simulink model "animation"  (R2023b)
settings: Solver=VariableStepAuto  StartTime=0.0  StopTime=30  RelTol=1e-3
libraries: vrlib x3, simulink x1
settings Model: Creator=tinas  LastModifiedBy=tinas

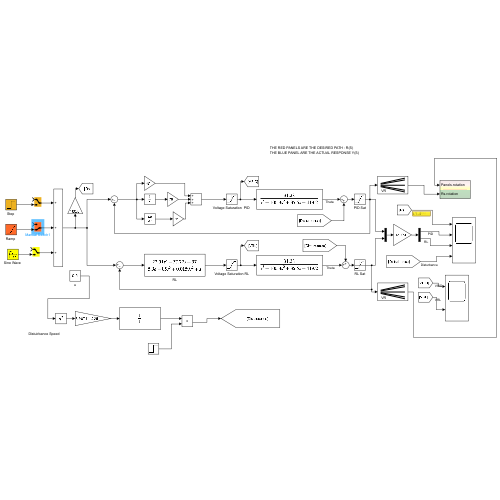
[thumbnail: Simulink's stored preview of the top-level diagram]
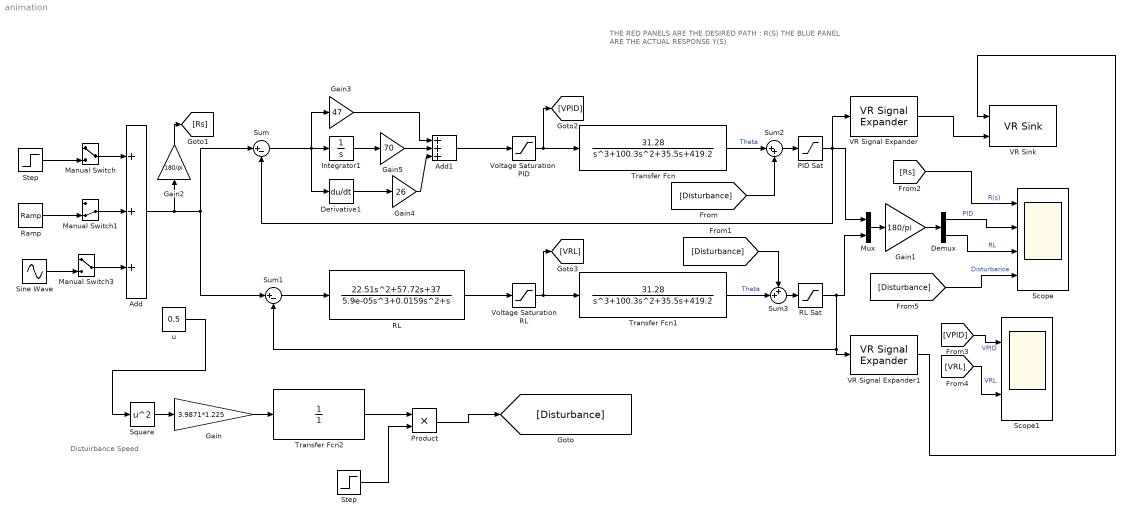
== system animation ==
  note: Distuirbance Speed
  note: THE RED PANELS ARE THE DESIRED PATH : R(S)
      | THE BLUE PANEL ARE THE ACTUAL RESPONSE Y(S)
  Add : Sum  Inputs=+++
  Add1 : Sum  Inputs=+++
  Demux : Demux  Outputs=2
  Derivative1 : Derivative
  Gain : Gain  Gain=3.9871*1.225
  Gain1 : Gain  Gain=180/pi
  Gain2 : Gain  Gain=180/pi
  Gain3 : Gain  Gain=47
  Gain4 : Gain  Gain=26
  Gain5 : Gain  Gain=70
  Integrator1 : Integrator
  Manual Switch : ManualSwitch
  Manual Switch1 : ManualSwitch  CurrentSetting=0
  Manual Switch3 : ManualSwitch
  Mux : Mux  Inputs=2
  PID Sat : Saturate  UpperLimit=pi/2  LowerLimit=-pi/2
  Product : Product
  RL : TransferFcn  Numerator=[22.51 57.72 37 ]  Denominator="[5.9e-05  0.0159  1 0]"
  RL Sat : Saturate  UpperLimit=pi/2  LowerLimit=-pi/2
  "Ramp " : simulink/Sources/Ramp  slope=0.01  start=0  InitialOutput=0
  Scope : Scope  NumInputPorts=4
  Scope1 : Scope  NumInputPorts=2
  "Sine Wave " : Sin  Amplitude=pi/2  SampleTime=0
  Square : Math  Operator=square
  Step : Step  Time=10  SampleTime=0
  "Step " : Step  Time=0  After=45*pi/180  SampleTime=0
  Sum : Sum  Inputs=|+-
  Sum1 : Sum  Inputs=|+-
  Sum2 : Sum  Inputs=|++
  Sum3 : Sum  Inputs=++|
  Transfer Fcn : TransferFcn  Numerator=[31.28]  Denominator="[1 100.3  35.5 419.2]"
  Transfer Fcn1 : TransferFcn  Numerator=[31.28]  Denominator="[1 100.3  35.5 419.2]"
  Transfer Fcn2 : TransferFcn  Denominator=[1]
  VR Signal Expander : vrlib/VR Signal Expander  outwidth=4  outidx=[4]
  VR Signal Expander1 : vrlib/VR Signal Expander  outwidth=4  outidx=[4]
  VR Sink : vrlib/VR Sink  InstantiateOnLoad=on  SampleTime=0.1  ViewEnable=on  RemoteChange=off  RemoteView=off  FieldsWritten=Panels.rotation.4.1.1.double#Rs.rotation.4.1.1.double  WorldFileName=Solar_Tracker.x3d  AutoView=off  VideoDimensions=[]  AllowVariableSize=off  FigureProperties="{'Position', 'Name', 'Viewpoint', 'CameraBound', 'CameraDirection', 'CameraPosition', 'CameraUpVector', 'ZoomFactor', 'Antialiasing', 'Headlight', 'Lighting', 'NavPanel', 'Sound', 'StatusBar', 'Stereo3D', 'Stereo3DCameraOffset', 'Stereo3DHIT', 'ToolBar', 'Textures', 'Transparency', 'Triad', 'Wireframe', 'NavZones', 'NavMode', 'NavSpeed', 'CaptureFileFormat', 'CaptureFileName', 'Record2DCompressMethod', 'Record2DCompressQuality', 'Record2D', 'Record2DFileName', 'Record2DFPS'; [6.2900000000000000e+02  -4.5540000000000009e+02   5.7600000000000000e+02   3.5000000000000000e+02], '', '', 'on', [0.0000000000000000e+00   0.0000000000000000e+00  -1.0000000000000000e+00], [0.0000000000000000e+00   0.0000000000000000e+00   1.0000000000000000e+01], [0.0000000000000000e+00   1.0000000000000000e+00   0.0000000000000000e+00], [2.5937424601000023e+00], 'on', 'on', 'on', 'halfbar', 'on', 'on', 'off', [1.0000000149011612e-01], [0.0000000000000000e+00], 'on', 'on', 'on', 'none', 'off', 'off', 'fly', 'normal', 'tif', '%f_anim_%n.tif', 'auto', [7.5000000000000000e+01], 'off', '%f_anim_%n.avi', 'auto'}"
  "Voltage Saturation  PID " : Saturate  UpperLimit=230  LowerLimit=-230
  Voltage Saturation RL : Saturate  UpperLimit=230  LowerLimit=-230
  u : Constant  Value=0.5
  wires:
  "Sine Wave "/1 -> Manual Switch3/2
  "Step "/1 -> Manual Switch/2
  Manual Switch3/1 -> Add/3
  Manual Switch1/1 -> Add/2
  "Ramp "/1 -> Manual Switch1/2
  Manual Switch/1 -> Add/1
  Add/1 -> Gain2/1, Sum1/1, Sum/1
  "Voltage Saturation  PID "/1 -> [VPID], Transfer Fcn/1
  Voltage Saturation RL/1 -> [VRL], Transfer Fcn1/1
  Add1/1 -> "Voltage Saturation  PID "/1
  Gain3/1 -> Add1/1
  Derivative1/1 -> Gain4/1
  Gain4/1 -> Add1/3
  Gain5/1 -> Add1/2
  Integrator1/1 -> Gain5/1
  Sum/1 -> Gain3/1, Derivative1/1, Integrator1/1
  RL/1 -> Voltage Saturation RL/1
  Sum1/1 -> RL/1
  u/1 -> Square/1
  Square/1 -> Gain/1
  Gain/1 -> Transfer Fcn2/1
  [Disturbance] -> Sum2/2
  [Disturbance] -> Sum3/1
  Mux/1 -> Gain1/1
  Gain2/1 -> [Rs]
  [Rs] -> Scope/1  "R(s)"
  Gain1/1 -> Demux/1
  Demux/1 -> Scope/2  "PID"
  Demux/2 -> Scope/3  "RL"
  [VRL] -> Scope1/2  "VRL"
  [VPID] -> Scope1/1  "VPID"
  [Disturbance] -> Scope/4  "Disturbance"
  Transfer Fcn2/1 -> Product/1
  Step/1 -> Product/2
  Product/1 -> [Disturbance]
  Transfer Fcn/1 -> Sum2/1  "Theta"
  Sum2/1 -> PID Sat/1
  PID Sat/1 -> VR Signal Expander/1, Sum/2, Mux/1
  Transfer Fcn1/1 -> Sum3/2  "Theta"
  Sum3/1 -> RL Sat/1
  RL Sat/1 -> VR Signal Expander1/1, Sum1/2, Mux/2
  VR Signal Expander/1 -> VR Sink/2
  VR Signal Expander1/1 -> VR Sink/1
